simulink library "halin"  (R2021b)
settings: Solver=VariableStepAuto  StartTime=0.0  StopTime=10.0  RelTol=1e-3
undefined symbols (not defined in the file): TRUE
libraries: FVT_lib x177, hcu_lib x55
(part 10 of 17)

== system halin/HAL_IN/CAN4/DKC1 ==
  DT_CAN4_SG_DKC1 : Inport
  DKCKeyNumSta : Subsystem
  DKCKeyTypeSta : Subsystem
  DKCPDkeyAreaRAPSSta : Subsystem
  DKCParkingModeCmd : Subsystem
  DKCReVehData : Subsystem
  PCommandToBCM : Subsystem
  PCommandToPTG : Subsystem
  PDKeyAreaLockUnlock : Subsystem
  PDKeyAreaPS : Subsystem
  PDKeyAreaPTG : Subsystem
  PDKeyWelcome : Subsystem
  PDkeyShowIVI : Subsystem
  PKeyMiss : Subsystem
  PKeyMode : Subsystem
  PUIDLowPower : Subsystem
  bus_selector : BusSelector  OutputSignals=CAN4_DKC_KeyNum_Sta
  bus_selector1 : BusSelector  OutputSignals=CAN4_DKC_KeyType_Sta
  bus_selector10 : BusSelector  OutputSignals=CAN4_P_DKey_Welcome
  bus_selector11 : BusSelector  OutputSignals=CAN4_P_Dkey_Show_IVI
  bus_selector12 : BusSelector  OutputSignals=CAN4_P_KeyMiss
  bus_selector13 : BusSelector  OutputSignals=CAN4_P_KeyMode
  bus_selector14 : BusSelector  OutputSignals=CAN4_P_UID_LowPower
  bus_selector2 : BusSelector  OutputSignals=CAN4_DKC_PDkeyAreaRAPS_Sta
  bus_selector3 : BusSelector  OutputSignals=CAN4_DKC_ParkingMode_Cmd
  bus_selector4 : BusSelector  OutputSignals=CAN4_DKC_Re_VehData
  bus_selector5 : BusSelector  OutputSignals=CAN4_P_CommandToBCM
  bus_selector6 : BusSelector  OutputSignals=CAN4_P_CommandToPTG
  bus_selector7 : BusSelector  OutputSignals=CAN4_P_DKey_Area_LockUnlock
  bus_selector8 : BusSelector  OutputSignals=CAN4_P_DKey_Area_PS
  bus_selector9 : BusSelector  OutputSignals=CAN4_P_DKey_Area_PTG
  VHAL_DKCKeyNumSta_enum : Outport
  VHAL_DKCKeyTypeSta_enum : Outport  Port=2
  VHAL_DKCPDkeyAreaRAPSSta_enum : Outport  Port=3
  VHAL_DKCParkingModeCmd_enum : Outport  Port=4
  VHAL_DKCReVehData_enum : Outport  Port=5
  VHAL_PCommandToBCM_enum : Outport  Port=6
  VHAL_PCommandToPTG_enum : Outport  Port=7
  VHAL_PDKeyAreaLockUnlock_enum : Outport  Port=8
  VHAL_PDKeyAreaPS_enum : Outport  Port=9
  VHAL_PDKeyAreaPTG_enum : Outport  Port=10
  VHAL_PDKeyWelcome_enum : Outport  Port=11
  VHAL_PDkeyShowIVI_enum : Outport  Port=12
  VHAL_PKeyMiss_flg : Outport  Port=13
  VHAL_PKeyMode_enum : Outport  Port=14
  VHAL_PUIDLowPower_flg : Outport  Port=15
  wires:
  DT_CAN4_SG_DKC1/1 -> [DT_CAN4_SG_DKC1]
  [DT_CAN4_SG_DKC1] -> bus_selector/1
  bus_selector/1 -> DKCKeyNumSta/1(DKC_KeyNum_Sta)  "<CAN4_DKC_KeyNum_Sta>"
  DKCKeyNumSta/1(VHAL_DKCKeyNumSta_enum) -> VHAL_DKCKeyNumSta_enum/1
  [DT_CAN4_SG_DKC1] -> bus_selector1/1
  bus_selector1/1 -> DKCKeyTypeSta/1(DKC_KeyType_Sta)  "<CAN4_DKC_KeyType_Sta>"
  DKCKeyTypeSta/1(VHAL_DKCKeyTypeSta_enum) -> VHAL_DKCKeyTypeSta_enum/1
  [DT_CAN4_SG_DKC1] -> bus_selector2/1
  bus_selector2/1 -> DKCPDkeyAreaRAPSSta/1(DKC_PDkeyAreaRAPS_Sta)  "<CAN4_DKC_PDkeyAreaRAPS_Sta>"
  DKCPDkeyAreaRAPSSta/1(VHAL_DKCPDkeyAreaRAPSSta_enum) -> VHAL_DKCPDkeyAreaRAPSSta_enum/1
  [DT_CAN4_SG_DKC1] -> bus_selector3/1
  bus_selector3/1 -> DKCParkingModeCmd/1(DKC_ParkingMode_Cmd)  "<CAN4_DKC_ParkingMode_Cmd>"
  DKCParkingModeCmd/1(VHAL_DKCParkingModeCmd_enum) -> VHAL_DKCParkingModeCmd_enum/1
  [DT_CAN4_SG_DKC1] -> bus_selector4/1
  bus_selector4/1 -> DKCReVehData/1(DKC_Re_VehData)  "<CAN4_DKC_Re_VehData>"
  DKCReVehData/1(VHAL_DKCReVehData_enum) -> VHAL_DKCReVehData_enum/1
  [DT_CAN4_SG_DKC1] -> bus_selector5/1
  bus_selector5/1 -> PCommandToBCM/1(P_CommandToBCM)  "<CAN4_P_CommandToBCM>"
  PCommandToBCM/1(VHAL_PCommandToBCM_enum) -> VHAL_PCommandToBCM_enum/1
  [DT_CAN4_SG_DKC1] -> bus_selector6/1
  bus_selector6/1 -> PCommandToPTG/1(P_CommandToPTG)  "<CAN4_P_CommandToPTG>"
  PCommandToPTG/1(VHAL_PCommandToPTG_enum) -> VHAL_PCommandToPTG_enum/1
  [DT_CAN4_SG_DKC1] -> bus_selector7/1
  bus_selector7/1 -> PDKeyAreaLockUnlock/1(P_DKey_Area_LockUnlock)  "<CAN4_P_DKey_Area_LockUnlock>"
  PDKeyAreaLockUnlock/1(VHAL_PDKeyAreaLockUnlock_enum) -> VHAL_PDKeyAreaLockUnlock_enum/1
  [DT_CAN4_SG_DKC1] -> bus_selector8/1
  bus_selector8/1 -> PDKeyAreaPS/1(P_DKey_Area_PS)  "<CAN4_P_DKey_Area_PS>"
  PDKeyAreaPS/1(VHAL_PDKeyAreaPS_enum) -> VHAL_PDKeyAreaPS_enum/1
  [DT_CAN4_SG_DKC1] -> bus_selector9/1
  bus_selector9/1 -> PDKeyAreaPTG/1(P_DKey_Area_PTG)  "<CAN4_P_DKey_Area_PTG>"
  PDKeyAreaPTG/1(VHAL_PDKeyAreaPTG_enum) -> VHAL_PDKeyAreaPTG_enum/1
  [DT_CAN4_SG_DKC1] -> bus_selector10/1
  bus_selector10/1 -> PDKeyWelcome/1(P_DKey_Welcome)  "<CAN4_P_DKey_Welcome>"
  PDKeyWelcome/1(VHAL_PDKeyWelcome_enum) -> VHAL_PDKeyWelcome_enum/1
  [DT_CAN4_SG_DKC1] -> bus_selector11/1
  bus_selector11/1 -> PDkeyShowIVI/1(P_Dkey_Show_IVI)  "<CAN4_P_Dkey_Show_IVI>"
  PDkeyShowIVI/1(VHAL_PDkeyShowIVI_enum) -> VHAL_PDkeyShowIVI_enum/1
  [DT_CAN4_SG_DKC1] -> bus_selector12/1
  bus_selector12/1 -> PKeyMiss/1(P_KeyMiss)  "<CAN4_P_KeyMiss>"
  PKeyMiss/1(VHAL_PKeyMiss_flg) -> VHAL_PKeyMiss_flg/1
  [DT_CAN4_SG_DKC1] -> bus_selector13/1
  bus_selector13/1 -> PKeyMode/1(P_KeyMode)  "<CAN4_P_KeyMode>"
  PKeyMode/1(VHAL_PKeyMode_enum) -> VHAL_PKeyMode_enum/1
  [DT_CAN4_SG_DKC1] -> bus_selector14/1
  bus_selector14/1 -> PUIDLowPower/1(P_UID_LowPower)  "<CAN4_P_UID_LowPower>"
  PUIDLowPower/1(VHAL_PUIDLowPower_flg) -> VHAL_PUIDLowPower_flg/1

== system halin/HAL_IN/CAN4/DKC2 ==
  DT_CAN4_SG_DKC2 : Inport
  EncryptionDATA063 : Subsystem
  EncryptionDATA64127 : Subsystem
  RandomNumberX : Subsystem
  bus_selector : BusSelector  OutputSignals=CAN4_EncryptionDATA_0_63
  bus_selector1 : BusSelector  OutputSignals=CAN4_EncryptionDATA_64_127
  bus_selector2 : BusSelector  OutputSignals=CAN4_Random_Number_X
  VHAL_EncryptionDATA063_enum : Outport
  VHAL_EncryptionDATA64127_enum : Outport  Port=2
  VHAL_RandomNumberX_enum : Outport  Port=3
  wires:
  DT_CAN4_SG_DKC2/1 -> [DT_CAN4_SG_DKC2]
  [DT_CAN4_SG_DKC2] -> bus_selector/1
  bus_selector/1 -> EncryptionDATA063/1(EncryptionDATA_0_63)  "<CAN4_EncryptionDATA_0_63>"
  EncryptionDATA063/1(VHAL_EncryptionDATA063_enum) -> VHAL_EncryptionDATA063_enum/1
  [DT_CAN4_SG_DKC2] -> bus_selector1/1
  bus_selector1/1 -> EncryptionDATA64127/1(EncryptionDATA_64_127)  "<CAN4_EncryptionDATA_64_127>"
  EncryptionDATA64127/1(VHAL_EncryptionDATA64127_enum) -> VHAL_EncryptionDATA64127_enum/1
  [DT_CAN4_SG_DKC2] -> bus_selector2/1
  bus_selector2/1 -> RandomNumberX/1(Random_Number_X)  "<CAN4_Random_Number_X>"
  RandomNumberX/1(VHAL_RandomNumberX_enum) -> VHAL_RandomNumberX_enum/1

== system halin/HAL_IN/CAN4/PTG1 ==
  DT_CAN4_SG_PTG1 : Inport
  PTGActiveSta : Subsystem
  PTGAutoStaus : Subsystem
  PTGExist : Subsystem
  PTGHWVer : Subsystem
  PTGInnerSW2 : Subsystem
  PTGIsSetHeight : Subsystem
  PTGRDILSta : Subsystem
  PTGSWVer : Subsystem
  PTGSysSta : Subsystem
  bus_selector : BusSelector  OutputSignals=CAN4_PTG_Active_Sta
  bus_selector1 : BusSelector  OutputSignals=CAN4_PTG_AutoStaus
  bus_selector2 : BusSelector  OutputSignals=CAN4_PTG_Exist
  bus_selector3 : BusSelector  OutputSignals=CAN4_PTG_HW_Ver
  bus_selector4 : BusSelector  OutputSignals=CAN4_PTG_Inner_SW_2
  bus_selector5 : BusSelector  OutputSignals=CAN4_PTG_Is_Set_Height
  bus_selector6 : BusSelector  OutputSignals=CAN4_PTG_RDIL_Sta
  bus_selector7 : BusSelector  OutputSignals=CAN4_PTG_SW_Ver
  bus_selector8 : BusSelector  OutputSignals=CAN4_PTG_Sys_Sta
  VHAL_PTGActiveSta_enum : Outport
  VHAL_PTGAutoStaus_flg : Outport  Port=2
  VHAL_PTGExist_flg : Outport  Port=3
  VHAL_PTGHWVer_enum : Outport  Port=4
  VHAL_PTGInnerSW2_enum : Outport  Port=5
  VHAL_PTGIsSetHeight_flg : Outport  Port=6
  VHAL_PTGRDILSta_enum : Outport  Port=7
  VHAL_PTGSWVer_enum : Outport  Port=8
  VHAL_PTGSysSta_enum : Outport  Port=9
  wires:
  DT_CAN4_SG_PTG1/1 -> [DT_CAN4_SG_PTG1]
  [DT_CAN4_SG_PTG1] -> bus_selector/1
  bus_selector/1 -> PTGActiveSta/1(PTG_Active_Sta)  "<CAN4_PTG_Active_Sta>"
  PTGActiveSta/1(VHAL_PTGActiveSta_enum) -> VHAL_PTGActiveSta_enum/1
  [DT_CAN4_SG_PTG1] -> bus_selector1/1
  bus_selector1/1 -> PTGAutoStaus/1(PTG_AutoStaus)  "<CAN4_PTG_AutoStaus>"
  PTGAutoStaus/1(VHAL_PTGAutoStaus_flg) -> VHAL_PTGAutoStaus_flg/1
  [DT_CAN4_SG_PTG1] -> bus_selector2/1
  bus_selector2/1 -> PTGExist/1(PTG_Exist)  "<CAN4_PTG_Exist>"
  PTGExist/1(VHAL_PTGExist_flg) -> VHAL_PTGExist_flg/1
  [DT_CAN4_SG_PTG1] -> bus_selector3/1
  bus_selector3/1 -> PTGHWVer/1(PTG_HW_Ver)  "<CAN4_PTG_HW_Ver>"
  PTGHWVer/1(VHAL_PTGHWVer_enum) -> VHAL_PTGHWVer_enum/1
  [DT_CAN4_SG_PTG1] -> bus_selector4/1
  bus_selector4/1 -> PTGInnerSW2/1(PTG_Inner_SW_2)  "<CAN4_PTG_Inner_SW_2>"
  PTGInnerSW2/1(VHAL_PTGInnerSW2_enum) -> VHAL_PTGInnerSW2_enum/1
  [DT_CAN4_SG_PTG1] -> bus_selector5/1
  bus_selector5/1 -> PTGIsSetHeight/1(PTG_Is_Set_Height)  "<CAN4_PTG_Is_Set_Height>"
  PTGIsSetHeight/1(VHAL_PTGIsSetHeight_flg) -> VHAL_PTGIsSetHeight_flg/1
  [DT_CAN4_SG_PTG1] -> bus_selector6/1
  bus_selector6/1 -> PTGRDILSta/1(PTG_RDIL_Sta)  "<CAN4_PTG_RDIL_Sta>"
  PTGRDILSta/1(VHAL_PTGRDILSta_enum) -> VHAL_PTGRDILSta_enum/1
  [DT_CAN4_SG_PTG1] -> bus_selector7/1
  bus_selector7/1 -> PTGSWVer/1(PTG_SW_Ver)  "<CAN4_PTG_SW_Ver>"
  PTGSWVer/1(VHAL_PTGSWVer_enum) -> VHAL_PTGSWVer_enum/1
  [DT_CAN4_SG_PTG1] -> bus_selector8/1
  bus_selector8/1 -> PTGSysSta/1(PTG_Sys_Sta)  "<CAN4_PTG_Sys_Sta>"
  PTGSysSta/1(VHAL_PTGSysSta_enum) -> VHAL_PTGSysSta_enum/1

== system halin/HAL_IN/CAN4/VHAL_CANMsgInvalidDKC1_flg ==
  Cast To Boolean13 : DataTypeConversion  OutDataTypeStr=boolean
  Constant : Constant  Value=TRUE
  Latch13 : hcu_lib/Basic_Blocks/Latch
  Switch13 : Switch  Criteria=u2 ~= 0
  Unit Delay : UnitDelay  SampleTime=-1  HasFrameUpgradeWarning=on
  UnitConverter : DataTypeConversion  OutDataTypeStr=boolean
  Out : Outport
  wires:
  Constant/1 -> Switch13/3
  Unit Delay/1 -> Cast To Boolean13/1
  Cast To Boolean13/1 -> Switch13/1, Latch13/1
  Switch13/1 -> UnitConverter/1
  Latch13/1 -> Switch13/2
  UnitConverter/1 -> Unit Delay/1, Out/1  "VHAL_CANMsgInvalidDKC1_flg"

== system halin/HAL_IN/CAN4/VHAL_CANMsgInvalidDKC2_flg ==
  Cast To Boolean13 : DataTypeConversion  OutDataTypeStr=boolean
  Constant : Constant  Value=TRUE
  Latch13 : hcu_lib/Basic_Blocks/Latch
  Switch13 : Switch  Criteria=u2 ~= 0
  Unit Delay : UnitDelay  SampleTime=-1  HasFrameUpgradeWarning=on
  UnitConverter : DataTypeConversion  OutDataTypeStr=boolean
  Out : Outport
  wires:
  Constant/1 -> Switch13/3
  Unit Delay/1 -> Cast To Boolean13/1
  Cast To Boolean13/1 -> Switch13/1, Latch13/1
  Switch13/1 -> UnitConverter/1
  Latch13/1 -> Switch13/2
  UnitConverter/1 -> Unit Delay/1, Out/1  "VHAL_CANMsgInvalidDKC2_flg"

== system halin/HAL_IN/CAN4/VHAL_CANMsgInvalidPTG1_flg ==
  Cast To Boolean13 : DataTypeConversion  OutDataTypeStr=boolean
  Constant : Constant  Value=TRUE
  Latch13 : hcu_lib/Basic_Blocks/Latch
  Switch13 : Switch  Criteria=u2 ~= 0
  Unit Delay : UnitDelay  SampleTime=-1  HasFrameUpgradeWarning=on
  UnitConverter : DataTypeConversion  OutDataTypeStr=boolean
  Out : Outport
  wires:
  Constant/1 -> Switch13/3
  Unit Delay/1 -> Cast To Boolean13/1
  Cast To Boolean13/1 -> Switch13/1, Latch13/1
  Switch13/1 -> UnitConverter/1
  Latch13/1 -> Switch13/2
  UnitConverter/1 -> Unit Delay/1, Out/1  "VHAL_CANMsgInvalidPTG1_flg"

== system halin/HAL_IN/CAN4/VHAL_CANMsgInvalidZONEDR1_flg ==
  Cast To Boolean13 : DataTypeConversion  OutDataTypeStr=boolean
  Constant : Constant  Value=TRUE
  Latch13 : hcu_lib/Basic_Blocks/Latch
  Switch13 : Switch  Criteria=u2 ~= 0
  Unit Delay : UnitDelay  SampleTime=-1  HasFrameUpgradeWarning=on
  UnitConverter : DataTypeConversion  OutDataTypeStr=boolean
  Out : Outport
  wires:
  Constant/1 -> Switch13/3
  Unit Delay/1 -> Cast To Boolean13/1
  Cast To Boolean13/1 -> Switch13/1, Latch13/1
  Switch13/1 -> UnitConverter/1
  Latch13/1 -> Switch13/2
  UnitConverter/1 -> Unit Delay/1, Out/1  "VHAL_CANMsgInvalidZONEDR1_flg"

== system halin/HAL_IN/CAN4/VHAL_CANMsgInvalidZONEDRVCU_flg ==
  Cast To Boolean13 : DataTypeConversion  OutDataTypeStr=boolean
  Constant : Constant  Value=TRUE
  Latch13 : hcu_lib/Basic_Blocks/Latch
  Switch13 : Switch  Criteria=u2 ~= 0
  Unit Delay : UnitDelay  SampleTime=-1  HasFrameUpgradeWarning=on
  UnitConverter : DataTypeConversion  OutDataTypeStr=boolean
  Out : Outport
  wires:
  Constant/1 -> Switch13/3
  Unit Delay/1 -> Cast To Boolean13/1
  Cast To Boolean13/1 -> Switch13/1, Latch13/1
  Switch13/1 -> UnitConverter/1
  Latch13/1 -> Switch13/2
  UnitConverter/1 -> Unit Delay/1, Out/1  "VHAL_CANMsgInvalidZONEDRVCU_flg"

== system halin/HAL_IN/CAN4/VHAL_CANMsgInvalidZONEFR1_flg ==
  Cast To Boolean13 : DataTypeConversion  OutDataTypeStr=boolean
  Constant : Constant  Value=TRUE
  Latch13 : hcu_lib/Basic_Blocks/Latch
  Switch13 : Switch  Criteria=u2 ~= 0
  Unit Delay : UnitDelay  SampleTime=-1  HasFrameUpgradeWarning=on
  UnitConverter : DataTypeConversion  OutDataTypeStr=boolean
  Out : Outport
  wires:
  Constant/1 -> Switch13/3
  Unit Delay/1 -> Cast To Boolean13/1
  Cast To Boolean13/1 -> Switch13/1, Latch13/1
  Switch13/1 -> UnitConverter/1
  Latch13/1 -> Switch13/2
  UnitConverter/1 -> Unit Delay/1, Out/1  "VHAL_CANMsgInvalidZONEFR1_flg"

== system halin/HAL_IN/CAN4/VHAL_CANMsgInvalidZONEFRVCU_flg ==
  Cast To Boolean13 : DataTypeConversion  OutDataTypeStr=boolean
  Constant : Constant  Value=TRUE
  Latch13 : hcu_lib/Basic_Blocks/Latch
  Switch13 : Switch  Criteria=u2 ~= 0
  Unit Delay : UnitDelay  SampleTime=-1  HasFrameUpgradeWarning=on
  UnitConverter : DataTypeConversion  OutDataTypeStr=boolean
  Out : Outport
  wires:
  Constant/1 -> Switch13/3
  Unit Delay/1 -> Cast To Boolean13/1
  Cast To Boolean13/1 -> Switch13/1, Latch13/1
  Switch13/1 -> UnitConverter/1
  Latch13/1 -> Switch13/2
  UnitConverter/1 -> Unit Delay/1, Out/1  "VHAL_CANMsgInvalidZONEFRVCU_flg"

== system halin/HAL_IN/CAN4/VHAL_CANMsgInvalidZONEL1_flg ==
  Cast To Boolean13 : DataTypeConversion  OutDataTypeStr=boolean
  Constant : Constant  Value=TRUE
  Latch13 : hcu_lib/Basic_Blocks/Latch
  Switch13 : Switch  Criteria=u2 ~= 0
  Unit Delay : UnitDelay  SampleTime=-1  HasFrameUpgradeWarning=on
  UnitConverter : DataTypeConversion  OutDataTypeStr=boolean
  Out : Outport
  wires:
  Constant/1 -> Switch13/3
  Unit Delay/1 -> Cast To Boolean13/1
  Cast To Boolean13/1 -> Switch13/1, Latch13/1
  Switch13/1 -> UnitConverter/1
  Latch13/1 -> Switch13/2
  UnitConverter/1 -> Unit Delay/1, Out/1  "VHAL_CANMsgInvalidZONEL1_flg"

== system halin/HAL_IN/CAN4/VHAL_CANMsgInvalidZONEL2_flg ==
  Cast To Boolean13 : DataTypeConversion  OutDataTypeStr=boolean
  Constant : Constant  Value=TRUE
  Latch13 : hcu_lib/Basic_Blocks/Latch
  Switch13 : Switch  Criteria=u2 ~= 0
  Unit Delay : UnitDelay  SampleTime=-1  HasFrameUpgradeWarning=on
  UnitConverter : DataTypeConversion  OutDataTypeStr=boolean
  Out : Outport
  wires:
  Constant/1 -> Switch13/3
  Unit Delay/1 -> Cast To Boolean13/1
  Cast To Boolean13/1 -> Switch13/1, Latch13/1
  Switch13/1 -> UnitConverter/1
  Latch13/1 -> Switch13/2
  UnitConverter/1 -> Unit Delay/1, Out/1  "VHAL_CANMsgInvalidZONEL2_flg"

== system halin/HAL_IN/CAN4/VHAL_CANMsgInvalidZONER1_flg ==
  Cast To Boolean13 : DataTypeConversion  OutDataTypeStr=boolean
  Constant : Constant  Value=TRUE
  Latch13 : hcu_lib/Basic_Blocks/Latch
  Switch13 : Switch  Criteria=u2 ~= 0
  Unit Delay : UnitDelay  SampleTime=-1  HasFrameUpgradeWarning=on
  UnitConverter : DataTypeConversion  OutDataTypeStr=boolean
  Out : Outport
  wires:
  Constant/1 -> Switch13/3
  Unit Delay/1 -> Cast To Boolean13/1
  Cast To Boolean13/1 -> Switch13/1, Latch13/1
  Switch13/1 -> UnitConverter/1
  Latch13/1 -> Switch13/2
  UnitConverter/1 -> Unit Delay/1, Out/1  "VHAL_CANMsgInvalidZONER1_flg"

== system halin/HAL_IN/CAN4/VHAL_CANMsgInvalidZONER2_flg ==
  Cast To Boolean13 : DataTypeConversion  OutDataTypeStr=boolean
  Constant : Constant  Value=TRUE
  Latch13 : hcu_lib/Basic_Blocks/Latch
  Switch13 : Switch  Criteria=u2 ~= 0
  Unit Delay : UnitDelay  SampleTime=-1  HasFrameUpgradeWarning=on
  UnitConverter : DataTypeConversion  OutDataTypeStr=boolean
  Out : Outport
  wires:
  Constant/1 -> Switch13/3
  Unit Delay/1 -> Cast To Boolean13/1
  Cast To Boolean13/1 -> Switch13/1, Latch13/1
  Switch13/1 -> UnitConverter/1
  Latch13/1 -> Switch13/2
  UnitConverter/1 -> Unit Delay/1, Out/1  "VHAL_CANMsgInvalidZONER2_flg"

== system halin/HAL_IN/CAN4/VHAL_CANMsgInvalidzGWAPTC1_flg ==
  Cast To Boolean13 : DataTypeConversion  OutDataTypeStr=boolean
  Constant : Constant  Value=TRUE
  Latch13 : hcu_lib/Basic_Blocks/Latch
  Switch13 : Switch  Criteria=u2 ~= 0
  Unit Delay : UnitDelay  SampleTime=-1  HasFrameUpgradeWarning=on
  UnitConverter : DataTypeConversion  OutDataTypeStr=boolean
  Out : Outport
  wires:
  Constant/1 -> Switch13/3
  Unit Delay/1 -> Cast To Boolean13/1
  Cast To Boolean13/1 -> Switch13/1, Latch13/1
  Switch13/1 -> UnitConverter/1
  Latch13/1 -> Switch13/2
  UnitConverter/1 -> Unit Delay/1, Out/1  "VHAL_CANMsgInvalidzGWAPTC1_flg"

== system halin/HAL_IN/CAN4/VHAL_CANMsgInvalidzGWCANFr1_flg ==
  Cast To Boolean13 : DataTypeConversion  OutDataTypeStr=boolean
  Constant : Constant  Value=TRUE
  Latch13 : hcu_lib/Basic_Blocks/Latch
  Switch13 : Switch  Criteria=u2 ~= 0
  Unit Delay : UnitDelay  SampleTime=-1  HasFrameUpgradeWarning=on
  UnitConverter : DataTypeConversion  OutDataTypeStr=boolean
  Out : Outport
  wires:
  Constant/1 -> Switch13/3
  Unit Delay/1 -> Cast To Boolean13/1
  Cast To Boolean13/1 -> Switch13/1, Latch13/1
  Switch13/1 -> UnitConverter/1
  Latch13/1 -> Switch13/2
  UnitConverter/1 -> Unit Delay/1, Out/1  "VHAL_CANMsgInvalidzGWCANFr1_flg"

== system halin/HAL_IN/CAN4/VHAL_CANMsgInvalidzGWLINDr1_flg ==
  Cast To Boolean13 : DataTypeConversion  OutDataTypeStr=boolean
  Constant : Constant  Value=TRUE
  Latch13 : hcu_lib/Basic_Blocks/Latch
  Switch13 : Switch  Criteria=u2 ~= 0
  Unit Delay : UnitDelay  SampleTime=-1  HasFrameUpgradeWarning=on
  UnitConverter : DataTypeConversion  OutDataTypeStr=boolean
  Out : Outport
  wires:
  Constant/1 -> Switch13/3
  Unit Delay/1 -> Cast To Boolean13/1
  Cast To Boolean13/1 -> Switch13/1, Latch13/1
  Switch13/1 -> UnitConverter/1
  Latch13/1 -> Switch13/2
  UnitConverter/1 -> Unit Delay/1, Out/1  "VHAL_CANMsgInvalidzGWLINDr1_flg"

== system halin/HAL_IN/CAN4/VHAL_CANMsgInvalidzGWLINFr1_flg ==
  Cast To Boolean13 : DataTypeConversion  OutDataTypeStr=boolean
  Constant : Constant  Value=TRUE
  Latch13 : hcu_lib/Basic_Blocks/Latch
  Switch13 : Switch  Criteria=u2 ~= 0
  Unit Delay : UnitDelay  SampleTime=-1  HasFrameUpgradeWarning=on
  UnitConverter : DataTypeConversion  OutDataTypeStr=boolean
  Out : Outport
  wires:
  Constant/1 -> Switch13/3
  Unit Delay/1 -> Cast To Boolean13/1
  Cast To Boolean13/1 -> Switch13/1, Latch13/1
  Switch13/1 -> UnitConverter/1
  Latch13/1 -> Switch13/2
  UnitConverter/1 -> Unit Delay/1, Out/1  "VHAL_CANMsgInvalidzGWLINFr1_flg"

== system halin/HAL_IN/CAN4/VHAL_CANMsgInvalidzGWSEAT1_flg ==
  Cast To Boolean13 : DataTypeConversion  OutDataTypeStr=boolean
  Constant : Constant  Value=TRUE
  Latch13 : hcu_lib/Basic_Blocks/Latch
  Switch13 : Switch  Criteria=u2 ~= 0
  Unit Delay : UnitDelay  SampleTime=-1  HasFrameUpgradeWarning=on
  UnitConverter : DataTypeConversion  OutDataTypeStr=boolean
  Out : Outport
  wires:
  Constant/1 -> Switch13/3
  Unit Delay/1 -> Cast To Boolean13/1
  Cast To Boolean13/1 -> Switch13/1, Latch13/1
  Switch13/1 -> UnitConverter/1
  Latch13/1 -> Switch13/2
  UnitConverter/1 -> Unit Delay/1, Out/1  "VHAL_CANMsgInvalidzGWSEAT1_flg"

== system halin/HAL_IN/CAN4/ZONE_DR1 ==
  DT_CAN4_SG_ZONE_DR1 : Inport
  DrLockSta : Subsystem
  MIRRORFOLDSW : Subsystem
  RLTurnLampC : Subsystem
  RRTurnLampC : Subsystem
  RWiperAS : Subsystem
  RWiperProtection : Subsystem
  bus_selector : BusSelector  OutputSignals=CAN4_DrLockSta
  bus_selector1 : BusSelector  OutputSignals=CAN4_MIRROR_FOLD_SW
  bus_selector2 : BusSelector  OutputSignals=CAN4_RLTurnLampC
  bus_selector3 : BusSelector  OutputSignals=CAN4_RRTurnLampC
  bus_selector4 : BusSelector  OutputSignals=CAN4_RWiperAS
  bus_selector5 : BusSelector  OutputSignals=CAN4_RWiperProtection
  VHAL_DrLockSta_flg : Outport
  VHAL_MIRRORFOLDSW_flg : Outport  Port=2
  VHAL_RLTurnLampC_mA : Outport  Port=3
  VHAL_RRTurnLampC_mA : Outport  Port=4
  VHAL_RWiperAS_flg : Outport  Port=5
  VHAL_RWiperProtection_flg : Outport  Port=6
  wires:
  DT_CAN4_SG_ZONE_DR1/1 -> [DT_CAN4_SG_ZONE_DR1]
  [DT_CAN4_SG_ZONE_DR1] -> bus_selector/1
  bus_selector/1 -> DrLockSta/1(DrLockSta)  "<CAN4_DrLockSta>"
  DrLockSta/1(VHAL_DrLockSta_flg) -> VHAL_DrLockSta_flg/1
  [DT_CAN4_SG_ZONE_DR1] -> bus_selector1/1
  bus_selector1/1 -> MIRRORFOLDSW/1(MIRROR_FOLD_SW)  "<CAN4_MIRROR_FOLD_SW>"
  MIRRORFOLDSW/1(VHAL_MIRRORFOLDSW_flg) -> VHAL_MIRRORFOLDSW_flg/1
  [DT_CAN4_SG_ZONE_DR1] -> bus_selector2/1
  bus_selector2/1 -> RLTurnLampC/1(RLTurnLampC)  "<CAN4_RLTurnLampC>"
  RLTurnLampC/1(VHAL_RLTurnLampC_mA) -> VHAL_RLTurnLampC_mA/1
  [DT_CAN4_SG_ZONE_DR1] -> bus_selector3/1
  bus_selector3/1 -> RRTurnLampC/1(RRTurnLampC)  "<CAN4_RRTurnLampC>"
  RRTurnLampC/1(VHAL_RRTurnLampC_mA) -> VHAL_RRTurnLampC_mA/1
  [DT_CAN4_SG_ZONE_DR1] -> bus_selector4/1
  bus_selector4/1 -> RWiperAS/1(RWiperAS)  "<CAN4_RWiperAS>"
  RWiperAS/1(VHAL_RWiperAS_flg) -> VHAL_RWiperAS_flg/1
  [DT_CAN4_SG_ZONE_DR1] -> bus_selector5/1
  bus_selector5/1 -> RWiperProtection/1(RWiperProtection)  "<CAN4_RWiperProtection>"
  RWiperProtection/1(VHAL_RWiperProtection_flg) -> VHAL_RWiperProtection_flg/1

== system halin/HAL_IN/CAN4/ZONE_DR_VCU ==
  DT_CAN4_SG_ZONE_DR_VCU : Inport
  BlowerErr : Subsystem
  DrPMMLVOutPErrLmp : Subsystem
  DrPMMSysErrLmp : Subsystem
  DrSCPSysErrLmp : Subsystem
  DrStdAErrSta : Subsystem
  SolarL : Subsystem
  SolarLErr : Subsystem
  SolarR : Subsystem
  SolarRErr : Subsystem
  TFaceL : Subsystem
  TFaceLErr : Subsystem
  TFaceR : Subsystem
  TFaceRErr : Subsystem
  TFaceRr : Subsystem
  TFaceRrErr : Subsystem
  TFootL : Subsystem
  TFootLErr : Subsystem
  TFootR : Subsystem
  TFootRErr : Subsystem
  TFootRr : Subsystem
  TFootRrErr : Subsystem
  Tevap : Subsystem
  TevapErr : Subsystem
  Tincar : Subsystem
  TincarErr : Subsystem
  ZoneDrMalfunLevel : Subsystem
  bus_selector : BusSelector  OutputSignals=CAN4_Blower_Err
  bus_selector1 : BusSelector  OutputSignals=CAN4_DrPMMLVOutPErrLmp
  bus_selector10 : BusSelector  OutputSignals=CAN4_T_Face_L_Err
  bus_selector11 : BusSelector  OutputSignals=CAN4_T_Face_R
  bus_selector12 : BusSelector  OutputSignals=CAN4_T_Face_R_Err
  bus_selector13 : BusSelector  OutputSignals=CAN4_T_Face_Rr
  bus_selector14 : BusSelector  OutputSignals=CAN4_T_Face_Rr_Err
  bus_selector15 : BusSelector  OutputSignals=CAN4_T_Foot_L
  bus_selector16 : BusSelector  OutputSignals=CAN4_T_Foot_L_Err
  bus_selector17 : BusSelector  OutputSignals=CAN4_T_Foot_R
  bus_selector18 : BusSelector  OutputSignals=CAN4_T_Foot_R_Err
  bus_selector19 : BusSelector  OutputSignals=CAN4_T_Foot_Rr
  bus_selector2 : BusSelector  OutputSignals=CAN4_DrPMMSysErrLmp
  bus_selector20 : BusSelector  OutputSignals=CAN4_T_Foot_Rr_Err
  bus_selector21 : BusSelector  OutputSignals=CAN4_Tevap
  bus_selector22 : BusSelector  OutputSignals=CAN4_Tevap_Err
  bus_selector23 : BusSelector  OutputSignals=CAN4_Tincar
  bus_selector24 : BusSelector  OutputSignals=CAN4_Tincar_Err
  bus_selector25 : BusSelector  OutputSignals=CAN4_ZoneDrMalfunLevel
  bus_selector3 : BusSelector  OutputSignals=CAN4_DrSCPSysErrLmp
  bus_selector4 : BusSelector  OutputSignals=CAN4_DrStdAErrSta
  bus_selector5 : BusSelector  OutputSignals=CAN4_SolarL
  bus_selector6 : BusSelector  OutputSignals=CAN4_SolarL_Err
  bus_selector7 : BusSelector  OutputSignals=CAN4_SolarR
  bus_selector8 : BusSelector  OutputSignals=CAN4_SolarR_Err
  bus_selector9 : BusSelector  OutputSignals=CAN4_T_Face_L
  VHAL_BlowerErr_enum : Outport
  VHAL_DrPMMLVOutPErrLmp_flg : Outport  Port=2
  VHAL_DrPMMSysErrLmp_flg : Outport  Port=3
  VHAL_DrSCPSysErrLmp_flg : Outport  Port=4
  VHAL_DrStdAErrSta_flg : Outport  Port=5
  VHAL_SolarL_W : Outport  Port=6
  VHAL_SolarLErr_enum : Outport  Port=7
  VHAL_SolarR_W : Outport  Port=8
  VHAL_SolarRErr_enum : Outport  Port=9
  VHAL_TFaceL_C : Outport  Port=10
  VHAL_TFaceLErr_enum : Outport  Port=11
  VHAL_TFaceR_C : Outport  Port=12
  VHAL_TFaceRErr_enum : Outport  Port=13
  VHAL_TFaceRr_C : Outport  Port=14
  VHAL_TFaceRrErr_enum : Outport  Port=15
  VHAL_TFootL_C : Outport  Port=16
  VHAL_TFootLErr_enum : Outport  Port=17
  VHAL_TFootR_C : Outport  Port=18
  VHAL_TFootRErr_enum : Outport  Port=19
  VHAL_TFootRr_C : Outport  Port=20
  VHAL_TFootRrErr_enum : Outport  Port=21
  VHAL_Tevap_C : Outport  Port=22
  VHAL_TevapErr_enum : Outport  Port=23
  VHAL_Tincar_C : Outport  Port=24
  VHAL_TincarErr_enum : Outport  Port=25
  VHAL_ZoneDrMalfunLevel_enum : Outport  Port=26
  wires:
  DT_CAN4_SG_ZONE_DR_VCU/1 -> [DT_CAN4_SG_ZONE_DR_VCU]
  [DT_CAN4_SG_ZONE_DR_VCU] -> bus_selector/1
  bus_selector/1 -> BlowerErr/1(Blower_Err)  "<CAN4_Blower_Err>"
  BlowerErr/1(VHAL_BlowerErr_enum) -> VHAL_BlowerErr_enum/1
  [DT_CAN4_SG_ZONE_DR_VCU] -> bus_selector1/1
  bus_selector1/1 -> DrPMMLVOutPErrLmp/1(DrPMMLVOutPErrLmp)  "<CAN4_DrPMMLVOutPErrLmp>"
  DrPMMLVOutPErrLmp/1(VHAL_DrPMMLVOutPErrLmp_flg) -> VHAL_DrPMMLVOutPErrLmp_flg/1
  [DT_CAN4_SG_ZONE_DR_VCU] -> bus_selector2/1
  bus_selector2/1 -> DrPMMSysErrLmp/1(DrPMMSysErrLmp)  "<CAN4_DrPMMSysErrLmp>"
  DrPMMSysErrLmp/1(VHAL_DrPMMSysErrLmp_flg) -> VHAL_DrPMMSysErrLmp_flg/1
  [DT_CAN4_SG_ZONE_DR_VCU] -> bus_selector3/1
  bus_selector3/1 -> DrSCPSysErrLmp/1(DrSCPSysErrLmp)  "<CAN4_DrSCPSysErrLmp>"
  DrSCPSysErrLmp/1(VHAL_DrSCPSysErrLmp_flg) -> VHAL_DrSCPSysErrLmp_flg/1
  [DT_CAN4_SG_ZONE_DR_VCU] -> bus_selector4/1
  bus_selector4/1 -> DrStdAErrSta/1(DrStdAErrSta)  "<CAN4_DrStdAErrSta>"
  DrStdAErrSta/1(VHAL_DrStdAErrSta_flg) -> VHAL_DrStdAErrSta_flg/1
  [DT_CAN4_SG_ZONE_DR_VCU] -> bus_selector5/1
  bus_selector5/1 -> SolarL/1(SolarL)  "<CAN4_SolarL>"
  SolarL/1(VHAL_SolarL_W) -> VHAL_SolarL_W/1
  [DT_CAN4_SG_ZONE_DR_VCU] -> bus_selector6/1
  bus_selector6/1 -> SolarLErr/1(SolarL_Err)  "<CAN4_SolarL_Err>"
  SolarLErr/1(VHAL_SolarLErr_enum) -> VHAL_SolarLErr_enum/1
  [DT_CAN4_SG_ZONE_DR_VCU] -> bus_selector7/1
  bus_selector7/1 -> SolarR/1(SolarR)  "<CAN4_SolarR>"
  SolarR/1(VHAL_SolarR_W) -> VHAL_SolarR_W/1
  [DT_CAN4_SG_ZONE_DR_VCU] -> bus_selector8/1
  bus_selector8/1 -> SolarRErr/1(SolarR_Err)  "<CAN4_SolarR_Err>"
  SolarRErr/1(VHAL_SolarRErr_enum) -> VHAL_SolarRErr_enum/1
  [DT_CAN4_SG_ZONE_DR_VCU] -> bus_selector9/1
  bus_selector9/1 -> TFaceL/1(T_Face_L)  "<CAN4_T_Face_L>"
  TFaceL/1(VHAL_TFaceL_C) -> VHAL_TFaceL_C/1
  [DT_CAN4_SG_ZONE_DR_VCU] -> bus_selector10/1
  bus_selector10/1 -> TFaceLErr/1(T_Face_L_Err)  "<CAN4_T_Face_L_Err>"
  TFaceLErr/1(VHAL_TFaceLErr_enum) -> VHAL_TFaceLErr_enum/1
  [DT_CAN4_SG_ZONE_DR_VCU] -> bus_selector11/1
  bus_selector11/1 -> TFaceR/1(T_Face_R)  "<CAN4_T_Face_R>"
  TFaceR/1(VHAL_TFaceR_C) -> VHAL_TFaceR_C/1
  [DT_CAN4_SG_ZONE_DR_VCU] -> bus_selector12/1
  bus_selector12/1 -> TFaceRErr/1(T_Face_R_Err)  "<CAN4_T_Face_R_Err>"
  TFaceRErr/1(VHAL_TFaceRErr_enum) -> VHAL_TFaceRErr_enum/1
  [DT_CAN4_SG_ZONE_DR_VCU] -> bus_selector13/1
  bus_selector13/1 -> TFaceRr/1(T_Face_Rr)  "<CAN4_T_Face_Rr>"
  TFaceRr/1(VHAL_TFaceRr_C) -> VHAL_TFaceRr_C/1
  [DT_CAN4_SG_ZONE_DR_VCU] -> bus_selector14/1
  bus_selector14/1 -> TFaceRrErr/1(T_Face_Rr_Err)  "<CAN4_T_Face_Rr_Err>"
  TFaceRrErr/1(VHAL_TFaceRrErr_enum) -> VHAL_TFaceRrErr_enum/1
  [DT_CAN4_SG_ZONE_DR_VCU] -> bus_selector15/1
  bus_selector15/1 -> TFootL/1(T_Foot_L)  "<CAN4_T_Foot_L>"
  TFootL/1(VHAL_TFootL_C) -> VHAL_TFootL_C/1
  [DT_CAN4_SG_ZONE_DR_VCU] -> bus_selector16/1
  bus_selector16/1 -> TFootLErr/1(T_Foot_L_Err)  "<CAN4_T_Foot_L_Err>"
  TFootLErr/1(VHAL_TFootLErr_enum) -> VHAL_TFootLErr_enum/1
  [DT_CAN4_SG_ZONE_DR_VCU] -> bus_selector17/1
  bus_selector17/1 -> TFootR/1(T_Foot_R)  "<CAN4_T_Foot_R>"
  TFootR/1(VHAL_TFootR_C) -> VHAL_TFootR_C/1
  [DT_CAN4_SG_ZONE_DR_VCU] -> bus_selector18/1
  bus_selector18/1 -> TFootRErr/1(T_Foot_R_Err)  "<CAN4_T_Foot_R_Err>"
  TFootRErr/1(VHAL_TFootRErr_enum) -> VHAL_TFootRErr_enum/1
  [DT_CAN4_SG_ZONE_DR_VCU] -> bus_selector19/1
  bus_selector19/1 -> TFootRr/1(T_Foot_Rr)  "<CAN4_T_Foot_Rr>"
  TFootRr/1(VHAL_TFootRr_C) -> VHAL_TFootRr_C/1
  [DT_CAN4_SG_ZONE_DR_VCU] -> bus_selector20/1
  bus_selector20/1 -> TFootRrErr/1(T_Foot_Rr_Err)  "<CAN4_T_Foot_Rr_Err>"
  TFootRrErr/1(VHAL_TFootRrErr_enum) -> VHAL_TFootRrErr_enum/1
  [DT_CAN4_SG_ZONE_DR_VCU] -> bus_selector21/1
  bus_selector21/1 -> Tevap/1(Tevap)  "<CAN4_Tevap>"
  Tevap/1(VHAL_Tevap_C) -> VHAL_Tevap_C/1
  [DT_CAN4_SG_ZONE_DR_VCU] -> bus_selector22/1
  bus_selector22/1 -> TevapErr/1(Tevap_Err)  "<CAN4_Tevap_Err>"
  TevapErr/1(VHAL_TevapErr_enum) -> VHAL_TevapErr_enum/1
  [DT_CAN4_SG_ZONE_DR_VCU] -> bus_selector23/1
  bus_selector23/1 -> Tincar/1(Tincar)  "<CAN4_Tincar>"
  Tincar/1(VHAL_Tincar_C) -> VHAL_Tincar_C/1
  [DT_CAN4_SG_ZONE_DR_VCU] -> bus_selector24/1
  bus_selector24/1 -> TincarErr/1(Tincar_Err)  "<CAN4_Tincar_Err>"
  TincarErr/1(VHAL_TincarErr_enum) -> VHAL_TincarErr_enum/1
  [DT_CAN4_SG_ZONE_DR_VCU] -> bus_selector25/1
  bus_selector25/1 -> ZoneDrMalfunLevel/1(ZoneDrMalfunLevel)  "<CAN4_ZoneDrMalfunLevel>"
  ZoneDrMalfunLevel/1(VHAL_ZoneDrMalfunLevel_enum) -> VHAL_ZoneDrMalfunLevel_enum/1

== system halin/HAL_IN/CAN4/ZONE_FR1 ==
  DT_CAN4_SG_ZONE_FR1 : Inport
  ChargeInletLockSta : Subsystem
  CompProEN : Subsystem
  FLTurnLampC : Subsystem
  FLTurnLightWarning : Subsystem
  FRTurnLampC : Subsystem
  FRTurnLightWarning : Subsystem
  FWiperAS : Subsystem
  FWiperProtection : Subsystem
  LADBHibeamIndication : Subsystem
  LADBOperationStatus : Subsystem
  LADBWarning : Subsystem
  LAHBWarning : Subsystem
  LDRLWarning : Subsystem
  LLBWarning : Subsystem
  LpositionLampWarning : Subsystem
  RADBHibeamIndication : Subsystem
  RADBOperationStatus : Subsystem
  RADBWarning : Subsystem
  RAHBWarning : Subsystem
  RDRLWarning : Subsystem
  RLBWarning : Subsystem
  RpositionLampWarning : Subsystem
  TrailerCheck : Subsystem
  TrailerModeSta : Subsystem
  ZFRBCMChargerDoorSWSta : Subsystem
  ZFRTHCMCLEVentActYSta : Subsystem
  ZFRTHCMCREVentActYSta : Subsystem
  ZFRTHCMDrEVentActYSta : Subsystem
  ZFRTHCMPsEVentActYSta : Subsystem
  bus_selector : BusSelector  OutputSignals=CAN4_ChargeInletLockSta
  bus_selector1 : BusSelector  OutputSignals=CAN4_CompProEN
  bus_selector10 : BusSelector  OutputSignals=CAN4_LADB_Warning
  bus_selector11 : BusSelector  OutputSignals=CAN4_LAHB_Warning
  bus_selector12 : BusSelector  OutputSignals=CAN4_LDRL_Warning
  bus_selector13 : BusSelector  OutputSignals=CAN4_LLB_Warning
  bus_selector14 : BusSelector  OutputSignals=CAN4_Lposition_Lamp_Warning
  bus_selector15 : BusSelector  OutputSignals=CAN4_RADB_Hibeam_Indication
  bus_selector16 : BusSelector  OutputSignals=CAN4_RADB_Operation_Status
  bus_selector17 : BusSelector  OutputSignals=CAN4_RADB_Warning
  bus_selector18 : BusSelector  OutputSignals=CAN4_RAHB_Warning
  bus_selector19 : BusSelector  OutputSignals=CAN4_RDRL_Warning
  bus_selector2 : BusSelector  OutputSignals=CAN4_FLTurnLampC
  bus_selector20 : BusSelector  OutputSignals=CAN4_RLB_Warning
  bus_selector21 : BusSelector  OutputSignals=CAN4_Rposition_Lamp_Warning
  bus_selector22 : BusSelector  OutputSignals=CAN4_TrailerCheck
  bus_selector23 : BusSelector  OutputSignals=CAN4_TrailerModeSta
  bus_selector24 : BusSelector  OutputSignals=CAN4_ZFR_BCM_ChargerDoorSW_Sta
  bus_selector25 : BusSelector  OutputSignals=CAN4_ZFR_THCM_CLEVentActY_Sta
  bus_selector26 : BusSelector  OutputSignals=CAN4_ZFR_THCM_CREVentActY_Sta
  bus_selector27 : BusSelector  OutputSignals=CAN4_ZFR_THCM_DrEVentActY_Sta
  bus_selector28 : BusSelector  OutputSignals=CAN4_ZFR_THCM_PsEVentActY_Sta
  bus_selector3 : BusSelector  OutputSignals=CAN4_FLTurn_Light_Warning
  bus_selector4 : BusSelector  OutputSignals=CAN4_FRTurnLampC
  bus_selector5 : BusSelector  OutputSignals=CAN4_FRTurn_Light_Warning
  bus_selector6 : BusSelector  OutputSignals=CAN4_FWiperAS
  bus_selector7 : BusSelector  OutputSignals=CAN4_FWiperProtection
  bus_selector8 : BusSelector  OutputSignals=CAN4_LADB_Hibeam_Indication
  bus_selector9 : BusSelector  OutputSignals=CAN4_LADB_Operation_Status
  VHAL_ChargeInletLockSta_flg : Outport
  VHAL_CompProEN_flg : Outport  Port=2
  VHAL_FLTurnLampC_mA : Outport  Port=3
  VHAL_FLTurnLightWarning_flg : Outport  Port=4
  VHAL_FRTurnLampC_mA : Outport  Port=5
  VHAL_FRTurnLightWarning_flg : Outport  Port=6
  VHAL_FWiperAS_flg : Outport  Port=7
  VHAL_FWiperProtection_flg : Outport  Port=8
  VHAL_LADBHibeamIndication_flg : Outport  Port=9
  VHAL_LADBOperationStatus_flg : Outport  Port=10
  VHAL_LADBWarning_flg : Outport  Port=11
  VHAL_LAHBWarning_flg : Outport  Port=12
  VHAL_LDRLWarning_flg : Outport  Port=13
  VHAL_LLBWarning_flg : Outport  Port=14
  VHAL_LpositionLampWarning_flg : Outport  Port=15
  VHAL_RADBHibeamIndication_flg : Outport  Port=16
  VHAL_RADBOperationStatus_flg : Outport  Port=17
  VHAL_RADBWarning_flg : Outport  Port=18
  VHAL_RAHBWarning_flg : Outport  Port=19
  VHAL_RDRLWarning_flg : Outport  Port=20
  VHAL_RLBWarning_flg : Outport  Port=21
  VHAL_RpositionLampWarning_flg : Outport  Port=22
  VHAL_TrailerCheck_flg : Outport  Port=23
  VHAL_TrailerModeSta_enum : Outport  Port=24
  VHAL_ZFRBCMChargerDoorSWSta_flg : Outport  Port=25
  VHAL_ZFRTHCMCLEVentActYSta_pct : Outport  Port=26
  VHAL_ZFRTHCMCREVentActYSta_pct : Outport  Port=27
  VHAL_ZFRTHCMDrEVentActYSta_pct : Outport  Port=28
  VHAL_ZFRTHCMPsEVentActYSta_pct : Outport  Port=29
  wires:
  DT_CAN4_SG_ZONE_FR1/1 -> [DT_CAN4_SG_ZONE_FR1]
  [DT_CAN4_SG_ZONE_FR1] -> bus_selector/1
  bus_selector/1 -> ChargeInletLockSta/1(ChargeInletLockSta)  "<CAN4_ChargeInletLockSta>"
  ChargeInletLockSta/1(VHAL_ChargeInletLockSta_flg) -> VHAL_ChargeInletLockSta_flg/1
  [DT_CAN4_SG_ZONE_FR1] -> bus_selector1/1
  bus_selector1/1 -> CompProEN/1(CompProEN)  "<CAN4_CompProEN>"
  CompProEN/1(VHAL_CompProEN_flg) -> VHAL_CompProEN_flg/1
  [DT_CAN4_SG_ZONE_FR1] -> bus_selector2/1
  bus_selector2/1 -> FLTurnLampC/1(FLTurnLampC)  "<CAN4_FLTurnLampC>"
  FLTurnLampC/1(VHAL_FLTurnLampC_mA) -> VHAL_FLTurnLampC_mA/1
  [DT_CAN4_SG_ZONE_FR1] -> bus_selector3/1
  bus_selector3/1 -> FLTurnLightWarning/1(FLTurn_Light_Warning)  "<CAN4_FLTurn_Light_Warning>"
  FLTurnLightWarning/1(VHAL_FLTurnLightWarning_flg) -> VHAL_FLTurnLightWarning_flg/1
  [DT_CAN4_SG_ZONE_FR1] -> bus_selector4/1
  bus_selector4/1 -> FRTurnLampC/1(FRTurnLampC)  "<CAN4_FRTurnLampC>"
  FRTurnLampC/1(VHAL_FRTurnLampC_mA) -> VHAL_FRTurnLampC_mA/1
  [DT_CAN4_SG_ZONE_FR1] -> bus_selector5/1
  bus_selector5/1 -> FRTurnLightWarning/1(FRTurn_Light_Warning)  "<CAN4_FRTurn_Light_Warning>"
  FRTurnLightWarning/1(VHAL_FRTurnLightWarning_flg) -> VHAL_FRTurnLightWarning_flg/1
  [DT_CAN4_SG_ZONE_FR1] -> bus_selector6/1
  bus_selector6/1 -> FWiperAS/1(FWiperAS)  "<CAN4_FWiperAS>"
  FWiperAS/1(VHAL_FWiperAS_flg) -> VHAL_FWiperAS_flg/1
  [DT_CAN4_SG_ZONE_FR1] -> bus_selector7/1
  bus_selector7/1 -> FWiperProtection/1(FWiperProtection)  "<CAN4_FWiperProtection>"
  FWiperProtection/1(VHAL_FWiperProtection_flg) -> VHAL_FWiperProtection_flg/1
  [DT_CAN4_SG_ZONE_FR1] -> bus_selector8/1
  bus_selector8/1 -> LADBHibeamIndication/1(LADB_Hibeam_Indication)  "<CAN4_LADB_Hibeam_Indication>"
  LADBHibeamIndication/1(VHAL_LADBHibeamIndication_flg) -> VHAL_LADBHibeamIndication_flg/1
  [DT_CAN4_SG_ZONE_FR1] -> bus_selector9/1
  bus_selector9/1 -> LADBOperationStatus/1(LADB_Operation_Status)  "<CAN4_LADB_Operation_Status>"
  LADBOperationStatus/1(VHAL_LADBOperationStatus_flg) -> VHAL_LADBOperationStatus_flg/1
  [DT_CAN4_SG_ZONE_FR1] -> bus_selector10/1
  bus_selector10/1 -> LADBWarning/1(LADB_Warning)  "<CAN4_LADB_Warning>"
  LADBWarning/1(VHAL_LADBWarning_flg) -> VHAL_LADBWarning_flg/1
  [DT_CAN4_SG_ZONE_FR1] -> bus_selector11/1
  bus_selector11/1 -> LAHBWarning/1(LAHB_Warning)  "<CAN4_LAHB_Warning>"
  LAHBWarning/1(VHAL_LAHBWarning_flg) -> VHAL_LAHBWarning_flg/1
  [DT_CAN4_SG_ZONE_FR1] -> bus_selector12/1
  bus_selector12/1 -> LDRLWarning/1(LDRL_Warning)  "<CAN4_LDRL_Warning>"
  LDRLWarning/1(VHAL_LDRLWarning_flg) -> VHAL_LDRLWarning_flg/1
  [DT_CAN4_SG_ZONE_FR1] -> bus_selector13/1
  bus_selector13/1 -> LLBWarning/1(LLB_Warning)  "<CAN4_LLB_Warning>"
  LLBWarning/1(VHAL_LLBWarning_flg) -> VHAL_LLBWarning_flg/1
  [DT_CAN4_SG_ZONE_FR1] -> bus_selector14/1
  bus_selector14/1 -> LpositionLampWarning/1(Lposition_Lamp_Warning)  "<CAN4_Lposition_Lamp_Warning>"
  LpositionLampWarning/1(VHAL_LpositionLampWarning_flg) -> VHAL_LpositionLampWarning_flg/1
  [DT_CAN4_SG_ZONE_FR1] -> bus_selector15/1
  bus_selector15/1 -> RADBHibeamIndication/1(RADB_Hibeam_Indication)  "<CAN4_RADB_Hibeam_Indication>"
  RADBHibeamIndication/1(VHAL_RADBHibeamIndication_flg) -> VHAL_RADBHibeamIndication_flg/1
  [DT_CAN4_SG_ZONE_FR1] -> bus_selector16/1
  bus_selector16/1 -> RADBOperationStatus/1(RADB_Operation_Status)  "<CAN4_RADB_Operation_Status>"
  RADBOperationStatus/1(VHAL_RADBOperationStatus_flg) -> VHAL_RADBOperationStatus_flg/1
  [DT_CAN4_SG_ZONE_FR1] -> bus_selector17/1
  bus_selector17/1 -> RADBWarning/1(RADB_Warning)  "<CAN4_RADB_Warning>"
  RADBWarning/1(VHAL_RADBWarning_flg) -> VHAL_RADBWarning_flg/1
  [DT_CAN4_SG_ZONE_FR1] -> bus_selector18/1
  bus_selector18/1 -> RAHBWarning/1(RAHB_Warning)  "<CAN4_RAHB_Warning>"
  RAHBWarning/1(VHAL_RAHBWarning_flg) -> VHAL_RAHBWarning_flg/1
  [DT_CAN4_SG_ZONE_FR1] -> bus_selector19/1
  bus_selector19/1 -> RDRLWarning/1(RDRL_Warning)  "<CAN4_RDRL_Warning>"
  RDRLWarning/1(VHAL_RDRLWarning_flg) -> VHAL_RDRLWarning_flg/1
  [DT_CAN4_SG_ZONE_FR1] -> bus_selector20/1
  bus_selector20/1 -> RLBWarning/1(RLB_Warning)  "<CAN4_RLB_Warning>"
  RLBWarning/1(VHAL_RLBWarning_flg) -> VHAL_RLBWarning_flg/1
  [DT_CAN4_SG_ZONE_FR1] -> bus_selector21/1
  bus_selector21/1 -> RpositionLampWarning/1(Rposition_Lamp_Warning)  "<CAN4_Rposition_Lamp_Warning>"
  RpositionLampWarning/1(VHAL_RpositionLampWarning_flg) -> VHAL_RpositionLampWarning_flg/1
  [DT_CAN4_SG_ZONE_FR1] -> bus_selector22/1
  bus_selector22/1 -> TrailerCheck/1(TrailerCheck)  "<CAN4_TrailerCheck>"
  TrailerCheck/1(VHAL_TrailerCheck_flg) -> VHAL_TrailerCheck_flg/1
  [DT_CAN4_SG_ZONE_FR1] -> bus_selector23/1
  bus_selector23/1 -> TrailerModeSta/1(TrailerModeSta)  "<CAN4_TrailerModeSta>"
  TrailerModeSta/1(VHAL_TrailerModeSta_enum) -> VHAL_TrailerModeSta_enum/1
  [DT_CAN4_SG_ZONE_FR1] -> bus_selector24/1
  bus_selector24/1 -> ZFRBCMChargerDoorSWSta/1(ZFR_BCM_ChargerDoorSW_Sta)  "<CAN4_ZFR_BCM_ChargerDoorSW_Sta>"
  ZFRBCMChargerDoorSWSta/1(VHAL_ZFRBCMChargerDoorSWSta_flg) -> VHAL_ZFRBCMChargerDoorSWSta_flg/1
  [DT_CAN4_SG_ZONE_FR1] -> bus_selector25/1
  bus_selector25/1 -> ZFRTHCMCLEVentActYSta/1(ZFR_THCM_CLEVentActY_Sta)  "<CAN4_ZFR_THCM_CLEVentActY_Sta>"
  ZFRTHCMCLEVentActYSta/1(VHAL_ZFRTHCMCLEVentActYSta_pct) -> VHAL_ZFRTHCMCLEVentActYSta_pct/1
  [DT_CAN4_SG_ZONE_FR1] -> bus_selector26/1
  bus_selector26/1 -> ZFRTHCMCREVentActYSta/1(ZFR_THCM_CREVentActY_Sta)  "<CAN4_ZFR_THCM_CREVentActY_Sta>"
  ZFRTHCMCREVentActYSta/1(VHAL_ZFRTHCMCREVentActYSta_pct) -> VHAL_ZFRTHCMCREVentActYSta_pct/1
  [DT_CAN4_SG_ZONE_FR1] -> bus_selector27/1
  bus_selector27/1 -> ZFRTHCMDrEVentActYSta/1(ZFR_THCM_DrEVentActY_Sta)  "<CAN4_ZFR_THCM_DrEVentActY_Sta>"
  ZFRTHCMDrEVentActYSta/1(VHAL_ZFRTHCMDrEVentActYSta_pct) -> VHAL_ZFRTHCMDrEVentActYSta_pct/1
  [DT_CAN4_SG_ZONE_FR1] -> bus_selector28/1
  bus_selector28/1 -> ZFRTHCMPsEVentActYSta/1(ZFR_THCM_PsEVentActY_Sta)  "<CAN4_ZFR_THCM_PsEVentActY_Sta>"
  ZFRTHCMPsEVentActYSta/1(VHAL_ZFRTHCMPsEVentActYSta_pct) -> VHAL_ZFRTHCMPsEVentActYSta_pct/1

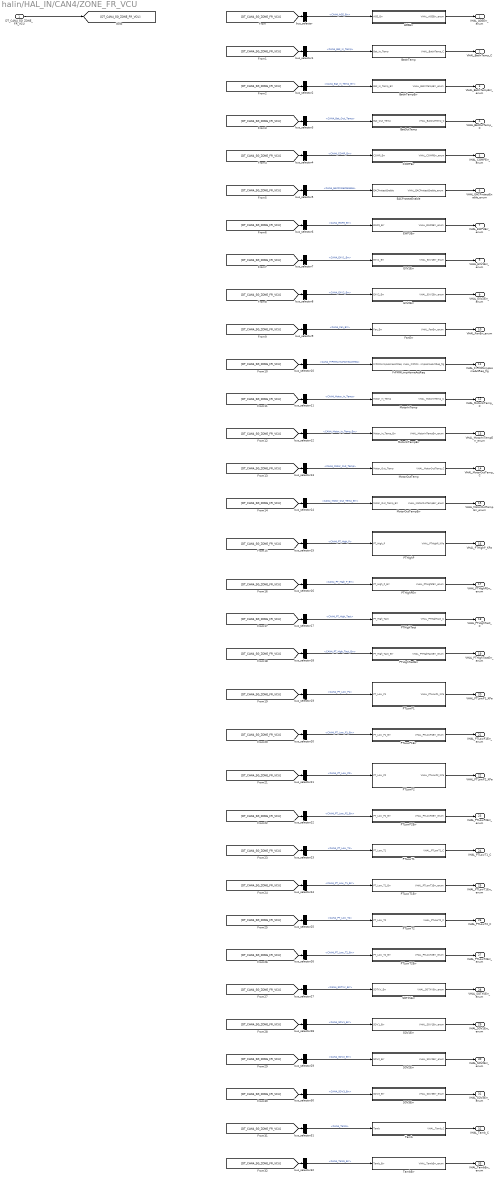
== system halin/HAL_IN/CAN4/ZONE_FR_VCU ==
  DT_CAN4_SG_ZONE_FR_VCU : Inport
  AGSErr : Subsystem
  BatInTemp : Subsystem
  BatInTempErr : Subsystem
  BatOutTemp : Subsystem
  COMPErr : Subsystem
  EACProtectEnable : Subsystem
  EWP3Err : Subsystem
  EXV1Err : Subsystem
  EXV2Err : Subsystem
  FanErr : Subsystem
  FrPMMLimpHomeActReq : Subsystem
  MotorInTemp : Subsystem
  MotorInTempErr : Subsystem
  MotorOutTemp : Subsystem
  MotorOutTempErr : Subsystem
  PTHighP : Subsystem
  PTHighPErr : Subsystem
  PTHighTact : Subsystem
  PTHighTactErr : Subsystem
  PTLowP1 : Subsystem
  PTLowP1Err : Subsystem
  PTLowP2 : Subsystem
  PTLowP2Err : Subsystem
  PTLowT1 : Subsystem
  PTLowT1Err : Subsystem
  PTLowT2 : Subsystem
  PTLowT2Err : Subsystem
  SOTXVErr : Subsystem
  SOV1Err : Subsystem
  SOV2Err : Subsystem
  SOV3Err : Subsystem
  Tamb : Subsystem
  TambErr : Subsystem
  bus_selector : BusSelector  OutputSignals=CAN4_AGS_Err
  bus_selector1 : BusSelector  OutputSignals=CAN4_Bat_In_Temp
  bus_selector10 : BusSelector  OutputSignals=CAN4_FrPMMLimpHomeActReq
  bus_selector11 : BusSelector  OutputSignals=CAN4_Motor_In_Temp
  bus_selector12 : BusSelector  OutputSignals=CAN4_Motor_In_Temp_Err
  bus_selector13 : BusSelector  OutputSignals=CAN4_Motor_Out_Temp
  bus_selector14 : BusSelector  OutputSignals=CAN4_Motor_Out_Temp_Err
  bus_selector15 : BusSelector  OutputSignals=CAN4_PT_High_P
  bus_selector16 : BusSelector  OutputSignals=CAN4_PT_High_P_Err
  bus_selector17 : BusSelector  OutputSignals=CAN4_PT_High_Tact
  bus_selector18 : BusSelector  OutputSignals=CAN4_PT_High_Tact_Err
  bus_selector19 : BusSelector  OutputSignals=CAN4_PT_Low_P1
  bus_selector2 : BusSelector  OutputSignals=CAN4_Bat_In_Temp_Err
  bus_selector20 : BusSelector  OutputSignals=CAN4_PT_Low_P1_Err
  bus_selector21 : BusSelector  OutputSignals=CAN4_PT_Low_P2
  bus_selector22 : BusSelector  OutputSignals=CAN4_PT_Low_P2_Err
  bus_selector23 : BusSelector  OutputSignals=CAN4_PT_Low_T1
  bus_selector24 : BusSelector  OutputSignals=CAN4_PT_Low_T1_Err
  bus_selector25 : BusSelector  OutputSignals=CAN4_PT_Low_T2
  bus_selector26 : BusSelector  OutputSignals=CAN4_PT_Low_T2_Err
  bus_selector27 : BusSelector  OutputSignals=CAN4_SOTXV_Err
  bus_selector28 : BusSelector  OutputSignals=CAN4_SOV1_Err
  bus_selector29 : BusSelector  OutputSignals=CAN4_SOV2_Err
  bus_selector3 : BusSelector  OutputSignals=CAN4_Bat_Out_Temp
  bus_selector30 : BusSelector  OutputSignals=CAN4_SOV3_Err
  bus_selector31 : BusSelector  OutputSignals=CAN4_Tamb
  bus_selector32 : BusSelector  OutputSignals=CAN4_Tamb_Err
  bus_selector4 : BusSelector  OutputSignals=CAN4_COMP_Err
  bus_selector5 : BusSelector  OutputSignals=CAN4_EACProtectEnable
  bus_selector6 : BusSelector  OutputSignals=CAN4_EWP3_Err
  bus_selector7 : BusSelector  OutputSignals=CAN4_EXV1_Err
  bus_selector8 : BusSelector  OutputSignals=CAN4_EXV2_Err
  bus_selector9 : BusSelector  OutputSignals=CAN4_Fan_Err
  VHAL_AGSErr_enum : Outport
  VHAL_BatInTemp_C : Outport  Port=2
  VHAL_BatInTempErr_enum : Outport  Port=3
  VHAL_BatOutTemp_C : Outport  Port=4
  VHAL_COMPErr_enum : Outport  Port=5
  VHAL_EACProtectEnable_enum : Outport  Port=6
  VHAL_EWP3Err_enum : Outport  Port=7
  VHAL_EXV1Err_enum : Outport  Port=8
  VHAL_EXV2Err_enum : Outport  Port=9
  VHAL_FanErr_enum : Outport  Port=10
  VHAL_FrPMMLimpHomeActReq_flg : Outport  Port=11
  VHAL_MotorInTemp_C : Outport  Port=12
  VHAL_MotorInTempErr_enum : Outport  Port=13
  VHAL_MotorOutTemp_C : Outport  Port=14
  VHAL_MotorOutTempErr_enum : Outport  Port=15
  VHAL_PTHighP_KPa : Outport  Port=16
  VHAL_PTHighPErr_enum : Outport  Port=17
  VHAL_PTHighTact_C : Outport  Port=18
  VHAL_PTHighTactErr_enum : Outport  Port=19
  VHAL_PTLowP1_KPa : Outport  Port=20
  VHAL_PTLowP1Err_enum : Outport  Port=21
  VHAL_PTLowP2_KPa : Outport  Port=22
  VHAL_PTLowP2Err_enum : Outport  Port=23
  VHAL_PTLowT1_C : Outport  Port=24
  VHAL_PTLowT1Err_enum : Outport  Port=25
  VHAL_PTLowT2_C : Outport  Port=26
  VHAL_PTLowT2Err_enum : Outport  Port=27
  VHAL_SOTXVErr_enum : Outport  Port=28
  VHAL_SOV1Err_enum : Outport  Port=29
  VHAL_SOV2Err_enum : Outport  Port=30
  VHAL_SOV3Err_enum : Outport  Port=31
  VHAL_Tamb_C : Outport  Port=32
  VHAL_TambErr_enum : Outport  Port=33
  wires:
  DT_CAN4_SG_ZONE_FR_VCU/1 -> [DT_CAN4_SG_ZONE_FR_VCU]
  [DT_CAN4_SG_ZONE_FR_VCU] -> bus_selector/1
  bus_selector/1 -> AGSErr/1(AGS_Err)  "<CAN4_AGS_Err>"
  AGSErr/1(VHAL_AGSErr_enum) -> VHAL_AGSErr_enum/1
  [DT_CAN4_SG_ZONE_FR_VCU] -> bus_selector1/1
  bus_selector1/1 -> BatInTemp/1(Bat_In_Temp)  "<CAN4_Bat_In_Temp>"
  BatInTemp/1(VHAL_BatInTemp_C) -> VHAL_BatInTemp_C/1
  [DT_CAN4_SG_ZONE_FR_VCU] -> bus_selector2/1
  bus_selector2/1 -> BatInTempErr/1(Bat_In_Temp_Err)  "<CAN4_Bat_In_Temp_Err>"
  BatInTempErr/1(VHAL_BatInTempErr_enum) -> VHAL_BatInTempErr_enum/1
  [DT_CAN4_SG_ZONE_FR_VCU] -> bus_selector3/1
  bus_selector3/1 -> BatOutTemp/1(Bat_Out_Temp)  "<CAN4_Bat_Out_Temp>"
  BatOutTemp/1(VHAL_BatOutTemp_C) -> VHAL_BatOutTemp_C/1
  [DT_CAN4_SG_ZONE_FR_VCU] -> bus_selector4/1
  bus_selector4/1 -> COMPErr/1(COMP_Err)  "<CAN4_COMP_Err>"
  COMPErr/1(VHAL_COMPErr_enum) -> VHAL_COMPErr_enum/1
  [DT_CAN4_SG_ZONE_FR_VCU] -> bus_selector5/1
  bus_selector5/1 -> EACProtectEnable/1(EACProtectEnable)  "<CAN4_EACProtectEnable>"
  EACProtectEnable/1(VHAL_EACProtectEnable_enum) -> VHAL_EACProtectEnable_enum/1
  [DT_CAN4_SG_ZONE_FR_VCU] -> bus_selector6/1
  bus_selector6/1 -> EWP3Err/1(EWP3_Err)  "<CAN4_EWP3_Err>"
  EWP3Err/1(VHAL_EWP3Err_enum) -> VHAL_EWP3Err_enum/1
  [DT_CAN4_SG_ZONE_FR_VCU] -> bus_selector7/1
  bus_selector7/1 -> EXV1Err/1(EXV1_Err)  "<CAN4_EXV1_Err>"
  EXV1Err/1(VHAL_EXV1Err_enum) -> VHAL_EXV1Err_enum/1
  [DT_CAN4_SG_ZONE_FR_VCU] -> bus_selector8/1
  bus_selector8/1 -> EXV2Err/1(EXV2_Err)  "<CAN4_EXV2_Err>"
  EXV2Err/1(VHAL_EXV2Err_enum) -> VHAL_EXV2Err_enum/1
  [DT_CAN4_SG_ZONE_FR_VCU] -> bus_selector9/1
  bus_selector9/1 -> FanErr/1(Fan_Err)  "<CAN4_Fan_Err>"
  FanErr/1(VHAL_FanErr_enum) -> VHAL_FanErr_enum/1
  [DT_CAN4_SG_ZONE_FR_VCU] -> bus_selector10/1
  bus_selector10/1 -> FrPMMLimpHomeActReq/1(FrPMMLimpHomeActReq)  "<CAN4_FrPMMLimpHomeActReq>"
  FrPMMLimpHomeActReq/1(VHAL_FrPMMLimpHomeActReq_flg) -> VHAL_FrPMMLimpHomeActReq_flg/1
  [DT_CAN4_SG_ZONE_FR_VCU] -> bus_selector11/1
  bus_selector11/1 -> MotorInTemp/1(Motor_In_Temp)  "<CAN4_Motor_In_Temp>"
  MotorInTemp/1(VHAL_MotorInTemp_C) -> VHAL_MotorInTemp_C/1
  [DT_CAN4_SG_ZONE_FR_VCU] -> bus_selector12/1
  bus_selector12/1 -> MotorInTempErr/1(Motor_In_Temp_Err)  "<CAN4_Motor_In_Temp_Err>"
  MotorInTempErr/1(VHAL_MotorInTempErr_enum) -> VHAL_MotorInTempErr_enum/1
  [DT_CAN4_SG_ZONE_FR_VCU] -> bus_selector13/1
  bus_selector13/1 -> MotorOutTemp/1(Motor_Out_Temp)  "<CAN4_Motor_Out_Temp>"
  MotorOutTemp/1(VHAL_MotorOutTemp_C) -> VHAL_MotorOutTemp_C/1
  [DT_CAN4_SG_ZONE_FR_VCU] -> bus_selector14/1
  bus_selector14/1 -> MotorOutTempErr/1(Motor_Out_Temp_Err)  "<CAN4_Motor_Out_Temp_Err>"
  MotorOutTempErr/1(VHAL_MotorOutTempErr_enum) -> VHAL_MotorOutTempErr_enum/1
  [DT_CAN4_SG_ZONE_FR_VCU] -> bus_selector15/1
  bus_selector15/1 -> PTHighP/1(PT_High_P)  "<CAN4_PT_High_P>"
  PTHighP/1(VHAL_PTHighP_KPa) -> VHAL_PTHighP_KPa/1
  [DT_CAN4_SG_ZONE_FR_VCU] -> bus_selector16/1
  bus_selector16/1 -> PTHighPErr/1(PT_High_P_Err)  "<CAN4_PT_High_P_Err>"
  PTHighPErr/1(VHAL_PTHighPErr_enum) -> VHAL_PTHighPErr_enum/1
  [DT_CAN4_SG_ZONE_FR_VCU] -> bus_selector17/1
  bus_selector17/1 -> PTHighTact/1(PT_High_Tact)  "<CAN4_PT_High_Tact>"
  PTHighTact/1(VHAL_PTHighTact_C) -> VHAL_PTHighTact_C/1
  [DT_CAN4_SG_ZONE_FR_VCU] -> bus_selector18/1
  bus_selector18/1 -> PTHighTactErr/1(PT_High_Tact_Err)  "<CAN4_PT_High_Tact_Err>"
  PTHighTactErr/1(VHAL_PTHighTactErr_enum) -> VHAL_PTHighTactErr_enum/1
  [DT_CAN4_SG_ZONE_FR_VCU] -> bus_selector19/1
  bus_selector19/1 -> PTLowP1/1(PT_Low_P1)  "<CAN4_PT_Low_P1>"
  PTLowP1/1(VHAL_PTLowP1_KPa) -> VHAL_PTLowP1_KPa/1
  [DT_CAN4_SG_ZONE_FR_VCU] -> bus_selector20/1
  bus_selector20/1 -> PTLowP1Err/1(PT_Low_P1_Err)  "<CAN4_PT_Low_P1_Err>"
  PTLowP1Err/1(VHAL_PTLowP1Err_enum) -> VHAL_PTLowP1Err_enum/1
  [DT_CAN4_SG_ZONE_FR_VCU] -> bus_selector21/1
  bus_selector21/1 -> PTLowP2/1(PT_Low_P2)  "<CAN4_PT_Low_P2>"
  PTLowP2/1(VHAL_PTLowP2_KPa) -> VHAL_PTLowP2_KPa/1
  [DT_CAN4_SG_ZONE_FR_VCU] -> bus_selector22/1
  bus_selector22/1 -> PTLowP2Err/1(PT_Low_P2_Err)  "<CAN4_PT_Low_P2_Err>"
  PTLowP2Err/1(VHAL_PTLowP2Err_enum) -> VHAL_PTLowP2Err_enum/1
  [DT_CAN4_SG_ZONE_FR_VCU] -> bus_selector23/1
  bus_selector23/1 -> PTLowT1/1(PT_Low_T1)  "<CAN4_PT_Low_T1>"
  PTLowT1/1(VHAL_PTLowT1_C) -> VHAL_PTLowT1_C/1
  [DT_CAN4_SG_ZONE_FR_VCU] -> bus_selector24/1
  bus_selector24/1 -> PTLowT1Err/1(PT_Low_T1_Err)  "<CAN4_PT_Low_T1_Err>"
  PTLowT1Err/1(VHAL_PTLowT1Err_enum) -> VHAL_PTLowT1Err_enum/1
  [DT_CAN4_SG_ZONE_FR_VCU] -> bus_selector25/1
  bus_selector25/1 -> PTLowT2/1(PT_Low_T2)  "<CAN4_PT_Low_T2>"
  PTLowT2/1(VHAL_PTLowT2_C) -> VHAL_PTLowT2_C/1
  [DT_CAN4_SG_ZONE_FR_VCU] -> bus_selector26/1
  bus_selector26/1 -> PTLowT2Err/1(PT_Low_T2_Err)  "<CAN4_PT_Low_T2_Err>"
  PTLowT2Err/1(VHAL_PTLowT2Err_enum) -> VHAL_PTLowT2Err_enum/1
  [DT_CAN4_SG_ZONE_FR_VCU] -> bus_selector27/1
  bus_selector27/1 -> SOTXVErr/1(SOTXV_Err)  "<CAN4_SOTXV_Err>"
  SOTXVErr/1(VHAL_SOTXVErr_enum) -> VHAL_SOTXVErr_enum/1
  [DT_CAN4_SG_ZONE_FR_VCU] -> bus_selector28/1
  bus_selector28/1 -> SOV1Err/1(SOV1_Err)  "<CAN4_SOV1_Err>"
  SOV1Err/1(VHAL_SOV1Err_enum) -> VHAL_SOV1Err_enum/1
  [DT_CAN4_SG_ZONE_FR_VCU] -> bus_selector29/1
  bus_selector29/1 -> SOV2Err/1(SOV2_Err)  "<CAN4_SOV2_Err>"
  SOV2Err/1(VHAL_SOV2Err_enum) -> VHAL_SOV2Err_enum/1
  [DT_CAN4_SG_ZONE_FR_VCU] -> bus_selector30/1
  bus_selector30/1 -> SOV3Err/1(SOV3_Err)  "<CAN4_SOV3_Err>"
  SOV3Err/1(VHAL_SOV3Err_enum) -> VHAL_SOV3Err_enum/1
  [DT_CAN4_SG_ZONE_FR_VCU] -> bus_selector31/1
  bus_selector31/1 -> Tamb/1(Tamb)  "<CAN4_Tamb>"
  Tamb/1(VHAL_Tamb_C) -> VHAL_Tamb_C/1
  [DT_CAN4_SG_ZONE_FR_VCU] -> bus_selector32/1
  bus_selector32/1 -> TambErr/1(Tamb_Err)  "<CAN4_Tamb_Err>"
  TambErr/1(VHAL_TambErr_enum) -> VHAL_TambErr_enum/1
